simulink model "PennyFab_Stochastic"  (R2015b)
settings: Solver=VariableStepDiscrete  StartTime=0.0  StopTime=5000  RelTol=1e-3
PostLoadFcn:
  | set_param(gcs, 'Location', [0 0 1500 750]);
InitFcn:
  | warning('off','all');
StartFcn:
  | warning('off','all');
libraries: simeventslib x3, simulink x1
CloseFcn:
  | warning('on','all');
Description:
  | % LICENSE:  3-clause "Revised" or "New" or "Modified" BSD License.
  | % Copyright (c) 2015, Georgia Institute of Technology.
  | % All rights reserved.
  | %
  | % Redistribution and use in source and binary forms, with or without
  | % modification, are permitted provided that the following conditions are met:
  | %     * Redistributions of source code must retain the above copyright
  | %       notice, this list of conditions and the following disclaimer.
  | %     * Redistributions in binary form must reproduce the above copyright
  | %       notice, this list of conditions and the following disclaimer in the
  | %       documentation and/or other materials provided with the distribution.
  | %     * Neither the name of the Georgia Institute of Technology nor the
  | %       names of its contributors may be used to endorse or promote products
  | %       derived from this software without specific prior written permission.
  | %
  | % THIS SOFTWARE IS PROVIDED BY THE COPYRIGHT HOLDERS AND CONTRIBUTORS "AS IS" AND
  | % ANY EXPRESS OR IMPLIED WARRANTIES, INCLUDING, BUT NOT LIMITED TO, THE IMPLIED
  | % WARRANTIES OF MERCHANTABILITY AND FITNESS FOR A PARTICULAR PURPOSE ARE
  | % DISCLAIMED. IN NO EVENT SHALL THE GEORGIA INSTITUTE OF TECHNOLOGY BE LIABLE FOR
  | % ANY DIRECT, INDIRECT, INCIDENTAL, SPECIAL, EXEMPLARY, OR CONSEQUENTIAL DAMAGES
  | % (INCLUDING, BUT NOT LIMITED TO, PROCUREMENT OF SUBSTITUTE GOODS OR SERVICES;
  | % LOSS OF USE, DATA, OR PROFITS; OR BUSINESS INTERRUPTION) HOWEVER CAUSED AND
  | % ON ANY THEORY OF LIABILITY, WHETHER IN CONTRACT, STRICT LIABILITY, OR TORT
  | % (INCLUDING NEGLIGENCE OR OTHERWISE) ARISING IN ANY WAY OUT OF THE USE OF THIS
  | % SOFTWARE, EVEN IF ADVISED OF THE POSSIBILITY OF SUCH DAMAGE.
settings Model: Creator=tsprock3  LastModifiedBy=tsprock3
settings DataIOCC: SaveFormat=Array
settings OptimizationCC: ExpressionDepthLimit=2147483647  SimCompilerOptimization=on
settings DebuggingCC: UnderspecifiedInitializationDetection=Classic  MergeDetectMultiDrivingBlocksExec=none  SolverPrmCheckMsg=warning  FcnCallInpInsideContextMsg=EnableAllAsWarning  StateNameClashWarn=warning
settings HardwareCC: ProdBitPerPointer=32  ProdLargestAtomicFloat=None  ProdIntDivRoundTo=Undefined  ProdEndianess=Unspecified  ProdWordSize=32  ProdHWDeviceType=32-bit Generic
settings GRTTargetCC: GeneratePreprocessorConditionals=Disable all
settings ConfigComp: CovModelRefEnable=Off

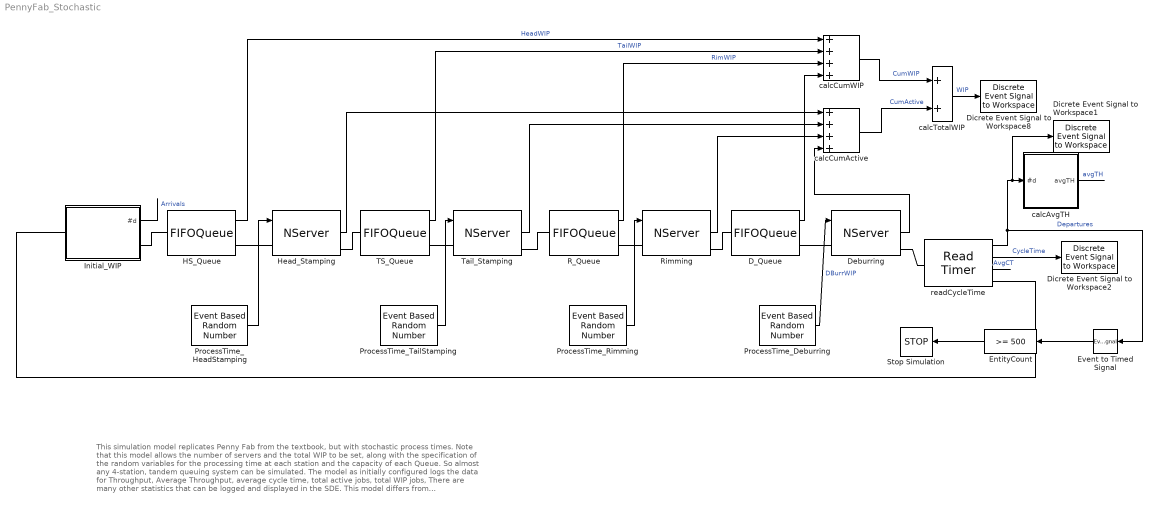
== system PennyFab_Stochastic ==
  note: This simulation model replicates Penny Fab from the textbook, but with stochastic process times.
      |
      | Note that this model allows the number of servers and the total WIP to be set, along with the specification of the random variables for the processing time at each station and the capacity of each Queue.  So almost any 4-station, tandem queuing system can be simulated.
      |
      | The model as initially configured logs the data for Throughput, Average Throughput, average cycle time, total active jobs, total WIP jobs, There are many other statistics that can be logged and displayed in the SDE.
      |
      | This model differs from PennyFab_Deterministic in another way--it includes the blocks necessary to compute the average throughput at every "completed" job.
  D_Queue : FIFOQueue  StatNumberInBlock=on
      settings: OutputPortMap=o1
  Deburring : NServer  NumberOfServers=2  ServiceTimeFrom=Signal port t  ServiceTime=2  StatNumberDeparted=on  StatNumberInBlock=on
      settings: OutputPortMap=o0,o1
  Dicrete Event Signal to Workspace1 : simeventslib/SimEvents Sinks/Discrete Event Signal to Workspace  VariableName=Departures  SaveFormat=Structure With Time  isMonitorOnly=off  isRecordIC=off
  Dicrete Event Signal to Workspace2 : simeventslib/SimEvents Sinks/Discrete Event Signal to Workspace  VariableName=CycleTime  SaveFormat=Structure With Time  isMonitorOnly=off  isRecordIC=off
  Dicrete Event Signal to Workspace8 : simeventslib/SimEvents Sinks/Discrete Event Signal to Workspace  VariableName=WIP  SaveFormat=Structure With Time  isMonitorOnly=off  isRecordIC=off
  EntityCount : simulink/Logic and Bit Operations/Compare To Constant  relop=>=  const=500  OutDataTypeStr=boolean
  Event to Timed Signal : EventToTimedSignal
  HS_Queue : FIFOQueue  StatNumberInBlock=on
      settings: OutputPortMap=o1
  Head_Stamping : NServer  NumberOfServers=1  ServiceTimeFrom=Signal port t  ServiceChange=Force complete  StatNumberDeparted=on  StatNumberInBlock=on
      settings: OutputPortMap=o0,o1
  Initial_WIP : Subsystem  mask{NumberOfEventsPerPeriod=25}
      mask prompts: NumberOfEventsPerPeriod "W =:  System WIP Level"
      mask TypeOptions NumberOfEventsPerPeriod: Generate/NumberOfEventsPerPeriod
      mask DialogControl DescTextVar Prompt: This parameter determines the total Work in Process (WIP) allowed in the closed system. The WIP level can impact the maximum throughput of the system.
  ProcessTime_Deburring : EventBasedRandomNumber  meanExp=3  minTri=.5  maxTri=5.5  modeTri=3  meanNorm=3  stdNorm=3  Seed=39663
  ProcessTime_HeadStamping : EventBasedRandomNumber  meanExp=2  minTri=.25  maxTri=4.75  modeTri=1  meanNorm=2  stdNorm=.33  Seed=42880
  ProcessTime_Rimming : EventBasedRandomNumber  meanExp=10  minTri=7  maxTri=13  modeTri=10  meanNorm=10  stdNorm=10  Seed=46097
  ProcessTime_TailStamping : EventBasedRandomNumber  meanExp=5  minTri=2  maxTri=8  modeTri=5  meanNorm=5  stdNorm=5  Seed=49314
  R_Queue : FIFOQueue  StatNumberInBlock=on
      settings: OutputPortMap=o1
  Rimming : NServer  NumberOfServers=6  ServiceTimeFrom=Signal port t  ServiceTime=6  StatNumberDeparted=on  StatNumberInBlock=on
      settings: OutputPortMap=o0,o1
  Stop Simulation : Stop
  TS_Queue : FIFOQueue  StatNumberInBlock=on
      settings: OutputPortMap=o1
  Tail_Stamping : NServer  NumberOfServers=2  ServiceTimeFrom=Signal port t  ServiceTime=2  StatNumberDeparted=on  StatNumberInBlock=on
      settings: OutputPortMap=o0,o1
  calcAvgTH : Subsystem
  calcCumActive : Sum  Inputs=4
  calcCumWIP : Sum  Inputs=4
  calcTotalWIP : Sum  Inputs=2
  readCycleTime : ReadTimer  TimerTag=CycleTime  StatNumberDeparted=on  StatTimeElapsed=on  StatAverageTimeElapsed=on
      settings: OutputPortMap=o0,o2,o3
  wires:
  ProcessTime_HeadStamping/1 -> Head_Stamping/1
  ProcessTime_TailStamping/1 -> Tail_Stamping/1
  ProcessTime_Rimming/1 -> Rimming/1
  HS_Queue/1 -> calcCumWIP/1  "HeadWIP"
  TS_Queue/1 -> calcCumWIP/2  "TailWIP"
  R_Queue/1 -> calcCumWIP/3  "RimWIP"
  ProcessTime_Deburring/1 -> Deburring/1  "DBurrWIP"
  calcCumWIP/1 -> calcTotalWIP/1  "CumWIP"
  D_Queue/1 -> calcCumWIP/4
  Rimming/2 -> calcCumActive/3
  Tail_Stamping/2 -> calcCumActive/2
  Head_Stamping/2 -> calcCumActive/1
  calcCumActive/1 -> calcTotalWIP/2  "CumActive"
  Deburring/2 -> calcCumActive/4
  readCycleTime/1 -> Dicrete Event Signal to Workspace1/1, calcAvgTH/1(#d), Event to Timed Signal/1  "Departures"
  calcTotalWIP/1 -> Dicrete Event Signal to Workspace8/1  "WIP"
  calcAvgTH/1(avgTH) -> ?  "avgTH"
  readCycleTime/2 -> Dicrete Event Signal to Workspace2/1  "CycleTime"
  readCycleTime/3 -> ?  "AvgCT"
  Initial_WIP/1(#d) -> ?  "Arrivals"
  EntityCount/1 -> Stop Simulation/1
  Event to Timed Signal/1 -> EntityCount/1
  connections:
  Deburring/RConn1 -- readCycleTime/LConn1
  readCycleTime/RConn1 -- Initial_WIP/LConn1
  Head_Stamping/RConn1 -- TS_Queue/LConn1
  TS_Queue/RConn1 -- Tail_Stamping/LConn1
  Tail_Stamping/RConn1 -- R_Queue/LConn1
  R_Queue/RConn1 -- Rimming/LConn1
  Rimming/RConn1 -- D_Queue/LConn1
  D_Queue/RConn1 -- Deburring/LConn1
  Initial_WIP/RConn1 -- HS_Queue/LConn1
  HS_Queue/RConn1 -- Head_Stamping/LConn1

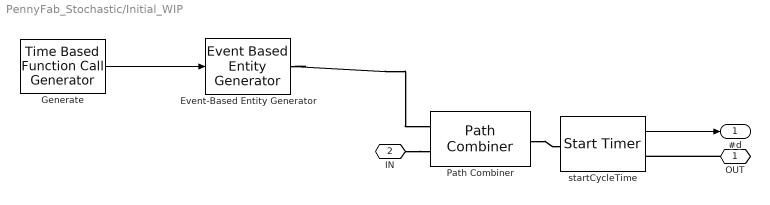
== system PennyFab_Stochastic/Initial_WIP ==
  Event-Based Entity Generator : EventBasedEntityGenerator  GenerateEntitiesUpon=Function call from port fcn
  Generate : TimeBasedFunctionCallGenerator  EventGenerationMode=Only at simulation start  NumberOfEventsPerPeriod=NumberOfEventsPerPeriod
  Path Combiner : PathCombiner  NumberInputPorts=2
  startCycleTime : StartTimer  TimerTag=CycleTime  TimerStartedOption=Restart  StatNumberDeparted=on
  OUT : PMIOPort  Port=1  Side=Right
  IN : PMIOPort  Port=2  Side=Left
  #d : Outport
  wires:
  Generate/1 -> Event-Based Entity Generator/1
  startCycleTime/1 -> #d/1
  connections:
  Path Combiner/RConn1 -- startCycleTime/LConn1
  OUT/RConn1 -- startCycleTime/RConn1
  IN/RConn1 -- Path Combiner/LConn2
  Event-Based Entity Generator/RConn1 -- Path Combiner/LConn1

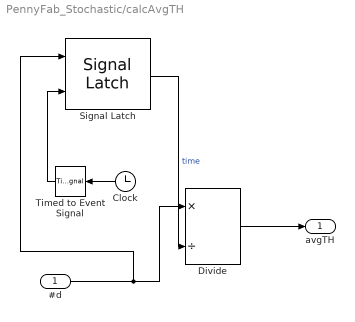
== system PennyFab_Stochastic/calcAvgTH ==
  #d : Inport
  Clock : Clock
  Divide : Product  Inputs=*/
  Signal Latch : SignalLatch  ReadMemoryUpon=Write to memory event
      settings: InputPortMap=u0,u2  OutputPortMap=o2
  Timed to Event Signal : TimedToEventSignal
  avgTH : Outport
  wires:
  #d/1 -> Signal Latch/1, Divide/1
  Timed to Event Signal/1 -> Signal Latch/2
  Signal Latch/1 -> Divide/2  "time"
  Clock/1 -> Timed to Event Signal/1
  Divide/1 -> avgTH/1
